simulink subsystem "WalkingRobotSubsystem"  (R2020a)
settings: Solver=VariableStepAuto  StartTime=0.0  StopTime=10.0  RelTol=1e-3
libraries: walkingRobotUtils x4, simulink x1
settings Model: Creator=brian  LastModifiedBy=brian

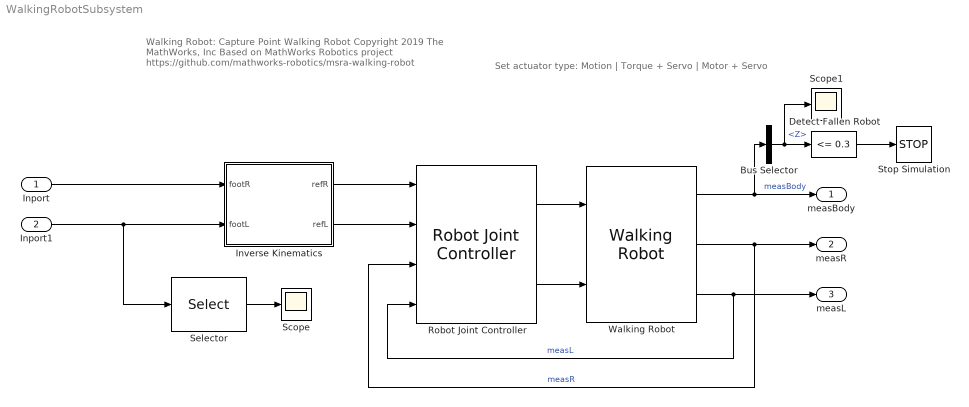
== system WalkingRobotSubsystem ==
  note: Walking Robot:
      | Capture Point Walking Robot
      | Copyright 2019 The MathWorks, Inc
      | Based on MathWorks Robotics project
      | https://github.com/mathworks-robotics/msra-walking-robot
  note: Set actuator type:
      | Motion | Torque + Servo | Motor + Servo
  Inport : Inport
  Inport1 : Inport  Port=2
  Bus Selector : BusSelector  OutputSignals=Z
  Detect Fallen Robot : simulink/Logic and Bit Operations/Compare To Constant  relop=<=  const=0.3  OutDataTypeStr=boolean
  Inverse Kinematics : Subsystem
  Robot Joint Controller : walkingRobotUtils/Robot Joint Controller  SystemSampleTime=-1  Latency=0  AutoFrameSizeCalculation=off
  Scope : Scope
  Scope1 : Scope
  Selector : Selector  NumberOfDimensions=2  InputPortWidth=3  IndexOptions=Index vector (dialog),Index vector (dialog)  Indices=[1,2,3],4  OutputSizes=1,1
  Stop Simulation : Stop
  Walking Robot : walkingRobotUtils/Walking Robot  SystemSampleTime=-1  Latency=0  AutoFrameSizeCalculation=off
  measBody : Outport  VectorParamsAs1DForOutWhenUnconnected=off
  measR : Outport  Port=2  VectorParamsAs1DForOutWhenUnconnected=off
  measL : Outport  Port=3  VectorParamsAs1DForOutWhenUnconnected=off
  wires:
  Inport1/1 -> Selector/1, Inverse Kinematics/2(footL)
  Detect Fallen Robot/1 -> Stop Simulation/1
  Inverse Kinematics/2(refL) -> Robot Joint Controller/2
  Inport/1 -> Inverse Kinematics/1(footR)
  Bus Selector/1 -> Scope1/1, Detect Fallen Robot/1  "<Z>"
  Selector/1 -> Scope/1
  Walking Robot/2 -> Robot Joint Controller/3, measR/1  "measR"
  Robot Joint Controller/2 -> Walking Robot/2
  Walking Robot/1 -> Bus Selector/1, measBody/1  "measBody"
  Robot Joint Controller/1 -> Walking Robot/1
  Inverse Kinematics/1(refR) -> Robot Joint Controller/1
  Walking Robot/3 -> Robot Joint Controller/4, measL/1  "measL"

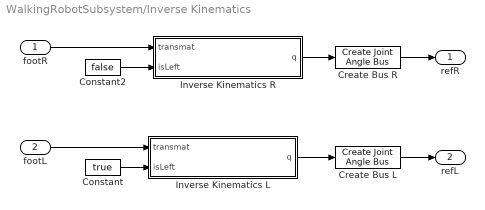
== system WalkingRobotSubsystem/Inverse Kinematics ==
  footR : Inport
  footL : Inport  Port=2
  Constant : Constant  Value=true
  Constant2 : Constant  Value=false
  Create Bus L : walkingRobotUtils/Create Joint Angle Bus  SystemSampleTime=-1  Latency=0  AutoFrameSizeCalculation=off
  Create Bus R : walkingRobotUtils/Create Joint Angle Bus  SystemSampleTime=-1  Latency=0  AutoFrameSizeCalculation=off
  Inverse Kinematics L : MATLAB Function  TreatAsAtomicUnit=on
  Inverse Kinematics R : MATLAB Function  TreatAsAtomicUnit=on
  refR : Outport
  refL : Outport  Port=2
  wires:
  footR/1 -> Inverse Kinematics R/1(transmat)
  Inverse Kinematics L/1(q) -> Create Bus L/1
  Constant2/1 -> Inverse Kinematics R/2(isLeft)
  Create Bus R/1 -> refR/1
  Create Bus L/1 -> refL/1
  Constant/1 -> Inverse Kinematics L/2(isLeft)
  Inverse Kinematics R/1(q) -> Create Bus R/1
  footL/1 -> Inverse Kinematics L/1(transmat)

== matlab function WalkingRobotSubsystem/Inverse Kinematics/Inverse Kinematics R ==
  data: transmat input; q output; isLeft input
function q = inverseKinematics(transmat, isLeft)
q = invKinBody2Foot(transmat, isLeft);

== matlab function WalkingRobotSubsystem/Inverse Kinematics/Inverse Kinematics L ==
  data: transmat input; q output; isLeft input
function q = inverseKinematics(transmat, isLeft)
q = invKinBody2Foot(transmat, isLeft);
